simulink model "Assignment_1"  (R2020b)
settings: Solver=VariableStepAuto  StartTime=0.0  StopTime=10.0  RelTol=1e-3
settings Model: Creator=Shantam Garg  LastModifiedBy=Shantam Garg

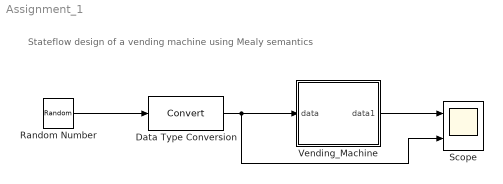
== system Assignment_1 ==
  note: Stateflow design of a vending machine using Mealy semantics
  Data Type Conversion : DataTypeConversion
  Random Number : RandomNumber  SampleTime=0.1
  Scope : Scope  NumInputPorts=2
  Vending_Machine : Stateflow chart  TreatAsAtomicUnit=on
  wires:
  Random Number/1 -> Data Type Conversion/1
  Data Type Conversion/1 -> Scope/2, Vending_Machine/1(data)
  Vending_Machine/1(data1) -> Scope/1

== stateflow chart Assignment_1/Vending_Machine ==
  data: data input; data1 output
